simulink model "Microstick_II_PlusDevBoard_33EP128MC202_Temperature_PIL_TOP"  (Simulink 7.9)
settings: Solver=FixedStepDiscrete  StartTime=0.0  StopTime=5  FixedStep=0.001  RelTol=1e-3
settings Model: Creator=Lubin Kerhuel  LastModifiedBy=Lubin Kerhuel
settings DataIOCC: LimitDataPoints=off  SaveFormat=StructureWithTime  SaveOutput=off  SignalLogging=off  DSMLogging=off  SaveTime=off
settings OptimizationCC: ExpressionDepthLimit=128  OptimizeModelRefInitCode=on  LifeSpan=Inf
settings DebuggingCC: StateNameClashWarn=none
settings HardwareCC: ProdBitPerInt=16  ProdBitPerPointer=16  ProdLargestAtomicInteger=Integer  ProdIntDivRoundTo=Zero  ProdEndianess=LittleEndian  ProdWordSize=16  ProdHWDeviceType=Generic->Custom
settings ModelReferenceCC: ModelReferenceNumInstancesAllowed=Single
settings RTWCC: SystemTargetFile=MCHP_dsPIC_stf.tlc  TemplateMakefile=MCHP_dsPIC.tmf  Description=Microchip Embedded Target PIC24 dsPIC30 dsPIC33 (real-time)  GenerateReport=on  ProcessScript=MCHP_dsPIC_stf_make_rtw_hook  IncludeHyperlinkInReport=on  GenerateTraceInfo=on  GenerateTraceReport=on  GenerateTraceReportSl=on  GenerateTraceReportSf=on  GenerateTraceReportEml=on
settings CodeAppCC: IgnoreCustomStorageClasses=off  MaxIdLength=255  CustomSymbolStrType=$N$R$M_T
settings STFCustomTargetCC: TargetLibSuffix=_lib.a  CodeReplacementLibrary=C89/C90 (ANSI)  CodeExecutionProfiling=on  IncludeMdlTerminateFcn=off  CombineOutputUpdateFcns=on  SuppressErrorStatus=on  ERTCustomFileBanners=on  SupportContinuousTime=off  GRTInterface=off  SystemTargetFile=MCHP_dsPIC_stf.tlc
settings ERTTargetCC: TargetLibSuffix=_lib.a  CodeReplacementLibrary=C89/C90 (ANSI)  CodeExecutionProfiling=on  MultiwordLength=2048  ParMdlRefBuildCompliant=off  CompOptLevelCompliant=off  ConcurrentExecutionCompliant=off  IncludeMdlTerminateFcn=off  SuppressErrorStatus=on  ERTFirstTimeCompliant=off  SupportNonInlinedSFcns=on  ModelStepFunctionPrototypeControlCompliant=off  CPPClassGenCompliant=off  CodeProfilingSaveOptions=AllData  ExtModeStaticAlloc=on  ExtModeStaticAllocSize=1  ExtModeMexFile=ext_serial_win32_comm_no_acks  ExtModeMexArgs=1 9 115200  ERTSrcFileBannerTemplate=MCHP_dsPIC_code_template.cgt  ERTHdrFileBannerTemplate=MCHP_dsPIC_code_template.cgt  ERTDataSrcFileTemplate=MCHP_dsPIC_code_template.cgt  ERTDataHdrFileTemplate=MCHP_dsPIC_code_template.cgt  ERTCustomFileTemplate=MCHP_main.tlc  ConvertIfToSwitch=off  SuppressUnreachableDefaultCases=off  CodeProfilingInstrumentation=on
settings CustomProperty: DataType=string  Value=33EP128MC202
settings EnumStrPairs: String=elf

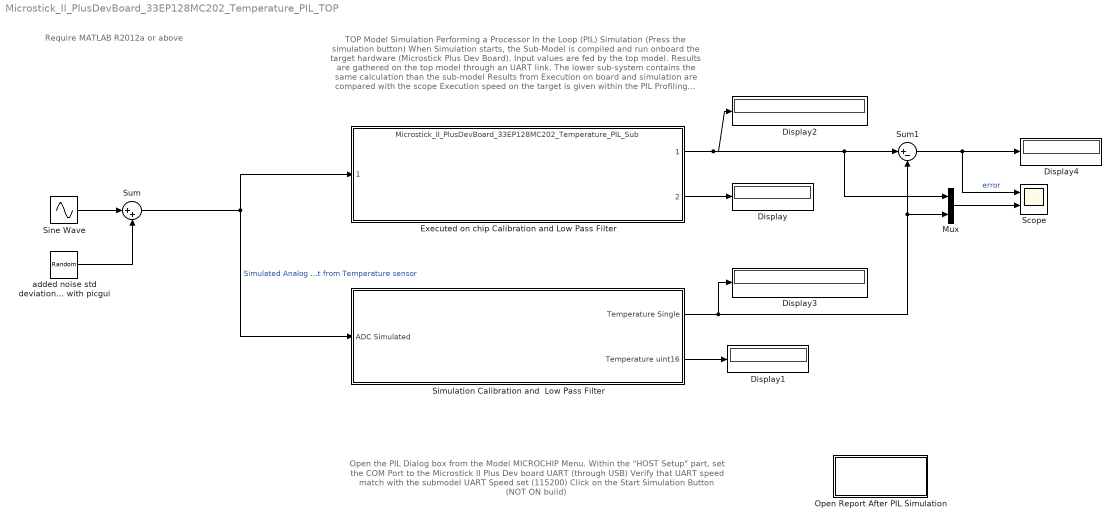
== system Microstick_II_PlusDevBoard_33EP128MC202_Temperature_PIL_TOP ==
  note: Open the PIL Dialog box from the Model MICROCHIP Menu.
      | Within the "HOST Setup" part, set the COM Port to the Microstick II Plus Dev board UART (through USB)
      | Verify that UART speed match with the submodel UART Speed set (115200)
      | Click on the Start Simulation Button (NOT ON build)
  note: TOP Model Simulation Performing a Processor In the Loop (PIL) Simulation (Press the simulation button)
      |
      | When Simulation starts, the Sub-Model is compiled and run onboard the target hardware (Microstick Plus Dev Board).
      | Input values are fed by the top model. Results are gathered on the top model through an UART link.
      | The lower sub-system contains the same calculation than the sub-model
      | Results from Execution on board and simulation are compared with the scope
      | Execution speed on the target is given within the PIL Profiling report.
  note: Require
      | MATLAB R2012a or above
  Display{,1..4} (5 alike) : Display
  Executed on chip Calibration and Low Pass Filter : ModelReference  ModelNameDialog=Microstick_II_PlusDevBoard_33EP128MC202_Temperature_PIL_Sub  SimulationMode=Processor-in-the-loop (PIL)  ModelReferenceVersion=1.236  CopyOfModelName=Microstick_II_PlusDevBoard_33EP128MC202_Temperature_PIL_Sub  DefaultDataLogging=on
  Mux : Mux  Inputs=2
  Open Report After PIL Simulation : Subsystem
      settings: OpenFcn=|
      | if exist('executionProfile','var') == 1
      | executionProfile.report;
      | else
      | errordlg('PIL has not run yet.', 'Run PIL first');
      | end
      mask Display: disp('Open PIL\nProfiling report');
  Scope : Scope  NumInputPorts=2
      settings: YMin=-1~24.13  YMax=1~24.36
  Simulation Calibration and  Low Pass Filter : Subsystem
  Sine Wave : Sin  Amplitude=50  Bias=14750  Frequency=2*pi  SampleTime=.001
  Sum : Sum  Inputs=|++  OutDataTypeStr=uint16  RndMeth=Round  SaturateOnIntegerOverflow=on
  Sum1 : Sum  Inputs=|+-
  added noise std deviation of raw values were measured with picgui : RandomNumber  Variance=2.5  SampleTime=0.001
  wires:
  Sine Wave/1 -> Sum/1
  added noise std deviation of raw values were measured with picgui/1 -> Sum/2
  Sum/1 -> Executed on chip Calibration and Low Pass Filter/1, Simulation Calibration and  Low Pass Filter/1(ADC Simulated)  "Simulated Analog output from Temperature sensor"
  Executed on chip Calibration and Low Pass Filter/2 -> Display/1
  Simulation Calibration and  Low Pass Filter/2(Temperature uint16) -> Display1/1
  Executed on chip Calibration and Low Pass Filter/1 -> Sum1/1, Mux/1, Display2/1
  Simulation Calibration and  Low Pass Filter/1(Temperature Single) -> Mux/2, Sum1/2, Display3/1
  Mux/1 -> Scope/2
  Sum1/1 -> Scope/1, Display4/1  "error"

== system Microstick_II_PlusDevBoard_33EP128MC202_Temperature_PIL_TOP/Open Report After PIL Simulation ==

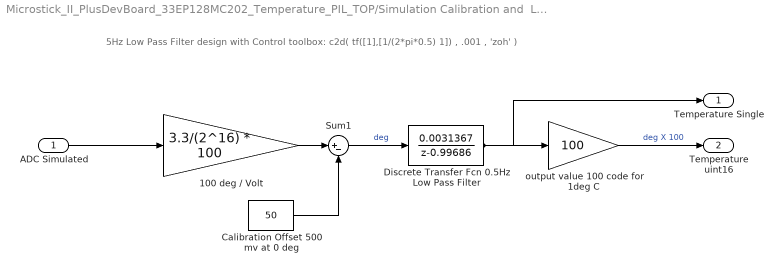
== system Microstick_II_PlusDevBoard_33EP128MC202_Temperature_PIL_TOP/Simulation Calibration and  Low Pass Filter ==
  note: 5Hz Low Pass Filter design with Control toolbox:
      | c2d( tf([1],[1/(2*pi*0.5) 1]) , .001 , 'zoh' )
  ADC Simulated : Inport  OutDataTypeStr=uint16  SampleTime=.001
  "100 deg / Volt " : Gain  Gain=3.3/(2^16) * 100  OutDataTypeStr=single
  Calibration Offset 500 mv at 0 deg : Constant  Value=50  OutDataTypeStr=Inherit: Inherit via back propagation  SampleTime=-1
  Discrete Transfer Fcn 0.5Hz Low Pass Filter : DiscreteTransferFcn  Numerator=[0.0031367]  Denominator=[1 -0.99686]
  Sum1 : Sum  Inputs=|+-
  output value 100 code for 1deg C : Gain  Gain=100  OutDataTypeStr=uint16
  Temperature Single : Outport  OutDataTypeStr=single  SampleTime=.001
  Temperature uint16 : Outport  Port=2  OutDataTypeStr=uint16  SampleTime=.001
  wires:
  Calibration Offset 500 mv at 0 deg/1 -> Sum1/2
  Sum1/1 -> Discrete Transfer Fcn 0.5Hz Low Pass Filter/1  "deg"
  Discrete Transfer Fcn 0.5Hz Low Pass Filter/1 -> output value 100 code for 1deg C/1, Temperature Single/1
  "100 deg / Volt "/1 -> Sum1/1
  output value 100 code for 1deg C/1 -> Temperature uint16/1  "deg X 100"
  ADC Simulated/1 -> "100 deg / Volt "/1
